simulink model "CF016A_GmVehSpdArbn"  (R2013b)
settings: Solver=FixedStepDiscrete  SolverMode=SingleTasking  StartTime=0.0  StopTime=1  FixedStep=0.002  RelTol=1e-3
undefined symbols (not defined in the file): DIAGCSTRTUPDLY_CNT_U32, NODEBSTEP_CNT_U16, NtcNr1, NtcSts1, VEHSPDMAX_KPH_F32
libraries: simulink x8, NxtrMax x7, NxtrMin x3, NxtrLim x3
(part 3 of 5)

== system CF016A_GmVehSpdArbn/GmVehSpdArbn/GmVehSpdArbnPer1/Calc_NTCIdleTi ==
  Constant1 : Constant  Value=DIAGCSTRTUPDLY_CNT_U32  OutDataTypeStr=uint32
  CopyRight2 : Subsystem  Description=|  mask(Copyright Information){none=on}
      | Copyright info block.                                               
      |                                                                     
      | Place copyright information at the top of every subsystem in design.
      mask prompts: none "No parameters"
      mask help: Place copyright information at the top of every subsystem in design.
      mask Display:
      | NxtrConf = 'Nexteer Confidential';
      | 
      | sys = bdroot; %handle for the current model ("system")
      | first = get_param(sys,'Created');
      | if(isempty(first))
      |     first = datestr(now,'yyyy');
      | else
      |     first = first(end-3:end);  %year is last four digits
      | end
      | 
      | last = get_param(sys,'LastModifiedDate');
      | if isempty(last)
      |     last = datestr(now,'yyyy');
      | else
      |     last = last(end-3:end);
      | end
      | 
      | if strcmp(first,last)
      |     fprintf('%s -- Copyright %s Nexteer',NxtrConf,first)
      | else
      |     fprintf('%s -- %s%s- %s Nexteer',NxtrConf,char(169),first,last)
      | end
  Data Store Read2 : DataStoreRead  DataStoreName=DiagcRefTi
  GetTiSpan100MicroSec32bit : Subsystem
  Relational Operator2 : RelationalOperator  Operator=>  OutDataTypeStr=boolean
  NTCIdleTiPassd : Outport
  wires:
  Constant1/1 -> Relational Operator2/2
  Relational Operator2/1 -> NTCIdleTiPassd/1  "NTCIdleTiPassd_Cnt_T_logl"
  Data Store Read2/1 -> GetTiSpan100MicroSec32bit/1(RefTmr)
  GetTiSpan100MicroSec32bit/1(TiSpan) -> Relational Operator2/1

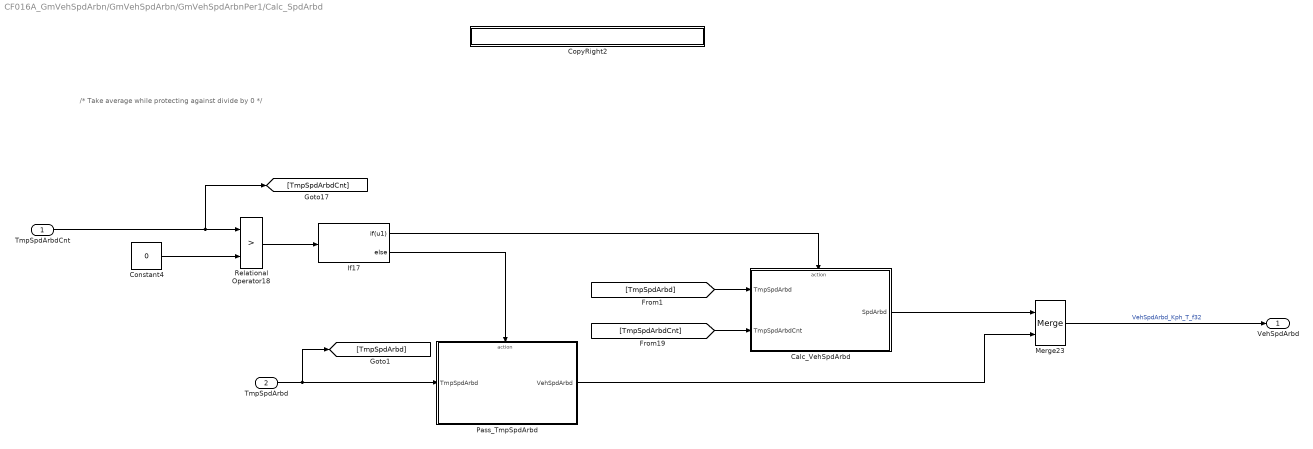
== system CF016A_GmVehSpdArbn/GmVehSpdArbn/GmVehSpdArbnPer1/Calc_SpdArbd ==
  note: /* Take average while protecting against divide by 0 */
  TmpSpdArbdCnt : Inport
  TmpSpdArbd : Inport  Port=2
  Calc_VehSpdArbd : Subsystem  TreatAsAtomicUnit=on
  Constant4 : Constant  Value=0  OutDataTypeStr=single
      settings: AttributesFormatString=%<OutDataTypeStr>
  CopyRight2 : Subsystem  Description=|  mask(Copyright Information){none=on}
      | Copyright info block.                                               
      |                                                                     
      | Place copyright information at the top of every subsystem in design.
      mask prompts: none "No parameters"
      mask help: Place copyright information at the top of every subsystem in design.
      mask Display:
      | NxtrConf = 'Nexteer Confidential';
      | 
      | sys = bdroot; %handle for the current model ("system")
      | first = get_param(sys,'Created');
      | if(isempty(first))
      |     first = datestr(now,'yyyy');
      | else
      |     first = first(end-3:end);  %year is last four digits
      | end
      | 
      | last = get_param(sys,'LastModifiedDate');
      | if isempty(last)
      |     last = datestr(now,'yyyy');
      | else
      |     last = last(end-3:end);
      | end
      | 
      | if strcmp(first,last)
      |     fprintf('%s -- Copyright %s Nexteer',NxtrConf,first)
      | else
      |     fprintf('%s -- %s%s- %s Nexteer',NxtrConf,char(169),first,last)
      | end
  If17 : If  IfExpression=u1
      settings: AttributesFormatString=%<Priority>
  Merge23 : Merge
  Pass_TmpSpdArbd : Subsystem  TreatAsAtomicUnit=on
  Relational Operator18 : RelationalOperator  Operator=>  OutDataTypeStr=boolean
  VehSpdArbd : Outport
  wires:
  Constant4/1 -> Relational Operator18/2
  Relational Operator18/1 -> If17/1
  If17/1 -> Calc_VehSpdArbd/Action
  If17/2 -> Pass_TmpSpdArbd/Action
  Pass_TmpSpdArbd/1(VehSpdArbd) -> Merge23/2
  Calc_VehSpdArbd/1(SpdArbd) -> Merge23/1
  Merge23/1 -> VehSpdArbd/1  "VehSpdArbd_Kph_T_f32"
  TmpSpdArbdCnt/1 -> [TmpSpdArbdCnt], Relational Operator18/1
  [TmpSpdArbdCnt] -> Calc_VehSpdArbd/2(TmpSpdArbdCnt)
  TmpSpdArbd/1 -> Pass_TmpSpdArbd/1(TmpSpdArbd), [TmpSpdArbd]
  [TmpSpdArbd] -> Calc_VehSpdArbd/1(TmpSpdArbd)

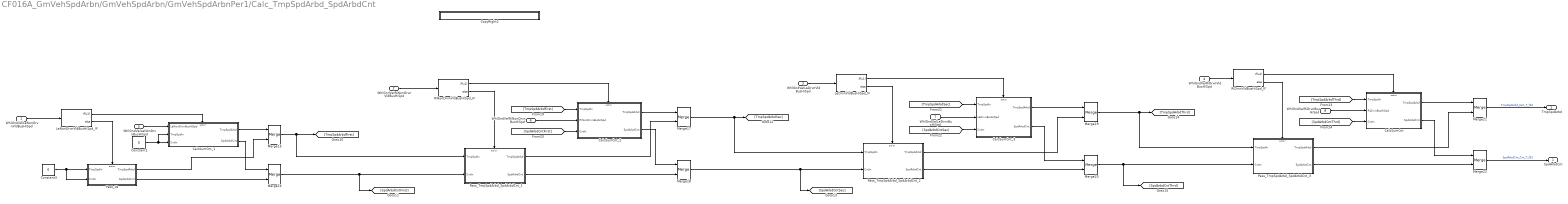
== system CF016A_GmVehSpdArbn/GmVehSpdArbn/GmVehSpdArbnPer1/Calc_TmpSpdArbd_SpdArbdCnt ==
  WhlGndVelLeNonDrvnVldBusHiSpd : Inport
  WhlGndVelRiNonDrvnVldBusHiSpd : Inport  RequirementInfo="{'linktype_rmi_doors' '0000c6e6 (/GM T1XX/SubSystem Specifications/Customer Functions/CF016A GM Vehicle Speed Arbitration)' '#197' 'true' 'REQ:  197' '' } %GIDa_75a6d6cd_4173_4b94_b70a_dd22fcf6fc32"  Port=2
  WhlGndVelLeDrvnVldBusHiSpd : Inport  RequirementInfo="{'linktype_rmi_doors' '0000c6e6 (/GM T1XX/SubSystem Specifications/Customer Functions/CF016A GM Vehicle Speed Arbitration)' '#197' 'true' 'REQ:  197' '' } %GIDa_bba5e7ef_449f_44f6_98d0_1ccf08468637"  Port=3
  WhlGndVelRiDrvnVldBusHiSpd : Inport  RequirementInfo="{'linktype_rmi_doors' '0000c6e6 (/GM T1XX/SubSystem Specifications/Customer Functions/CF016A GM Vehicle Speed Arbitration)' '#197' 'true' 'REQ:  197' '' } %GIDa_b5b50655_d2e5_4a4e_9d9c_e6104a63ae0b"  Port=4
  WhlGndVelLeNonDrvnBusHiSpd : Inport  RequirementInfo="{'linktype_rmi_doors' '0000c6e6 (/GM T1XX/SubSystem Specifications/Customer Functions/CF016A GM Vehicle Speed Arbitration)' '#197' 'true' 'REQ:  197' '' } %GIDa_3165a49e_7db2_44a5_86aa_6dde81cf1a65"  Port=5
  WhlGndVelRiNonDrvnBusHiSpd : Inport  RequirementInfo="{'linktype_rmi_doors' '0000c6e6 (/GM T1XX/SubSystem Specifications/Customer Functions/CF016A GM Vehicle Speed Arbitration)' '#197' 'true' 'REQ:  197' '' } %GIDa_3798149f_5af7_41c0_afc1_7eafa55e1dcf"  Port=6
  WhlGndVelLeDrvnBusHiSpd : Inport  RequirementInfo="{'linktype_rmi_doors' '0000c6e6 (/GM T1XX/SubSystem Specifications/Customer Functions/CF016A GM Vehicle Speed Arbitration)' '#197' 'true' 'REQ:  197' '' } %GIDa_8f8a555f_8d7e_4f96_a446_1dcec9e14b78"  Port=7
  WhlGndVelRiDrvnBusHiSpd : Inport  RequirementInfo="{'linktype_rmi_doors' '0000c6e6 (/GM T1XX/SubSystem Specifications/Customer Functions/CF016A GM Vehicle Speed Arbitration)' '#197' 'true' 'REQ:  197' '' } %GIDa_00fa1cd6_a6a5_410d_9383_797401eb3683"  Port=8
  CalcSumCnt : Subsystem  RequirementInfo="{'linktype_rmi_doors' '0000c6e6 (/GM T1XX/SubSystem Specifications/Customer Functions/CF016A GM Vehicle Speed Arbitration)' '#197' 'true' 'REQ:  197' '' } %GIDa_a224d60f_a880_4ee1_8319_45ce552737be"  TreatAsAtomicUnit=on
  CalcSumCnt_1 : Subsystem  RequirementInfo="{'linktype_rmi_doors' '0000c6e6 (/GM T1XX/SubSystem Specifications/Customer Functions/CF016A GM Vehicle Speed Arbitration)' '#197' 'true' 'REQ:  197' '' } %GIDa_a912f7bd_e18e_48b0_96ea_183fa55b44d1"  TreatAsAtomicUnit=on
  CalcSumCnt_2 : Subsystem  RequirementInfo="{'linktype_rmi_doors' '0000c6e6 (/GM T1XX/SubSystem Specifications/Customer Functions/CF016A GM Vehicle Speed Arbitration)' '#197' 'true' 'REQ:  197' '' } %GIDa_908d3886_164f_47bf_8eb5_d3c275cb63fb"  TreatAsAtomicUnit=on
  CalcSumCnt_3 : Subsystem  RequirementInfo="{'linktype_rmi_doors' '0000c6e6 (/GM T1XX/SubSystem Specifications/Customer Functions/CF016A GM Vehicle Speed Arbitration)' '#197' 'true' 'REQ:  197' '' } %GIDa_0cfda85e_115e_4a3a_86a7_df581f2b4836"  TreatAsAtomicUnit=on
  Constant1 : Constant  Value=0  OutDataTypeStr=single
      settings: AttributesFormatString=%<OutDataTypeStr>
  Constant3 : Constant  Value=0  OutDataTypeStr=single
      settings: AttributesFormatString=%<OutDataTypeStr>
  CopyRight2 : Subsystem  Description=|  mask(Copyright Information){none=on}
      | Copyright info block.                                               
      |                                                                     
      | Place copyright information at the top of every subsystem in design.
      mask prompts: none "No parameters"
      mask help: Place copyright information at the top of every subsystem in design.
      mask Display:
      | NxtrConf = 'Nexteer Confidential';
      | 
      | sys = bdroot; %handle for the current model ("system")
      | first = get_param(sys,'Created');
      | if(isempty(first))
      |     first = datestr(now,'yyyy');
      | else
      |     first = first(end-3:end);  %year is last four digits
      | end
      | 
      | last = get_param(sys,'LastModifiedDate');
      | if isempty(last)
      |     last = datestr(now,'yyyy');
      | else
      |     last = last(end-3:end);
      | end
      | 
      | if strcmp(first,last)
      |     fprintf('%s -- Copyright %s Nexteer',NxtrConf,first)
      | else
      |     fprintf('%s -- %s%s- %s Nexteer',NxtrConf,char(169),first,last)
      | end
  LeDrvnVldBusHiSpd_IF : If  RequirementInfo="{'linktype_rmi_doors' '0000c6e6 (/GM T1XX/SubSystem Specifications/Customer Functions/CF016A GM Vehicle Speed Arbitration)' '#197' 'true' 'REQ:  197' '' } %GIDa_e5398537_68ff_4ca3_873a_5860dedb4f38"  IfExpression=u1
      settings: AttributesFormatString=%<Priority>
  LeNonDrvnVldBusHiSpd_IF : If  RequirementInfo="{'linktype_rmi_doors' '0000c6e6 (/GM T1XX/SubSystem Specifications/Customer Functions/CF016A GM Vehicle Speed Arbitration)' '#197' 'true' 'REQ:  197' '' } %GIDa_0a5ef933_02c3_4017_8cbc_cbbf00c96bdb"  IfExpression=u1
      settings: AttributesFormatString=%<Priority>
  Merge15 : Merge  RequirementInfo="{'linktype_rmi_doors' '0000c6e6 (/GM T1XX/SubSystem Specifications/Customer Functions/CF016A GM Vehicle Speed Arbitration)' '#197' 'true' 'REQ:  197' '' } %GIDa_b01b27b6_2653_40db_b669_b9a443f48c3f"
  Merge16 : Merge  RequirementInfo="{'linktype_rmi_doors' '0000c6e6 (/GM T1XX/SubSystem Specifications/Customer Functions/CF016A GM Vehicle Speed Arbitration)' '#197' 'true' 'REQ:  197' '' } %GIDa_8a935c09_276b_472e_be93_82eb8a41092d"
  Merge17 : Merge  RequirementInfo="{'linktype_rmi_doors' '0000c6e6 (/GM T1XX/SubSystem Specifications/Customer Functions/CF016A GM Vehicle Speed Arbitration)' '#197' 'true' 'REQ:  197' '' } %GIDa_1a065b5b_19d5_4f28_8260_459213537fb4"
  Merge18 : Merge  RequirementInfo="{'linktype_rmi_doors' '0000c6e6 (/GM T1XX/SubSystem Specifications/Customer Functions/CF016A GM Vehicle Speed Arbitration)' '#197' 'true' 'REQ:  197' '' } %GIDa_74f763ca_8a5c_4a42_8005_2c77b166578e"
  Merge19 : Merge  RequirementInfo="{'linktype_rmi_doors' '0000c6e6 (/GM T1XX/SubSystem Specifications/Customer Functions/CF016A GM Vehicle Speed Arbitration)' '#197' 'true' 'REQ:  197' '' } %GIDa_3ff2a4ad_b1a8_4288_966c_4fbb914ab0f1"
  Merge20 : Merge  RequirementInfo="{'linktype_rmi_doors' '0000c6e6 (/GM T1XX/SubSystem Specifications/Customer Functions/CF016A GM Vehicle Speed Arbitration)' '#197' 'true' 'REQ:  197' '' } %GIDa_5cafa504_1ff8_4f3c_b0c4_59e13f736e29"
  Merge21 : Merge  RequirementInfo="{'linktype_rmi_doors' '0000c6e6 (/GM T1XX/SubSystem Specifications/Customer Functions/CF016A GM Vehicle Speed Arbitration)' '#197' 'true' 'REQ:  197' '' } %GIDa_e6f4a7a3_924e_49ec_a51b_ec7f1402c916"
  Merge22 : Merge  RequirementInfo="{'linktype_rmi_doors' '0000c6e6 (/GM T1XX/SubSystem Specifications/Customer Functions/CF016A GM Vehicle Speed Arbitration)' '#197' 'true' 'REQ:  197' '' } %GIDa_5f365e82_5eef_48d0_8df9_073c5a4821ae"
  Pass_0s : Subsystem  RequirementInfo="{'linktype_rmi_doors' '0000c6e6 (/GM T1XX/SubSystem Specifications/Customer Functions/CF016A GM Vehicle Speed Arbitration)' '#197' 'true' 'REQ:  197' '' } %GIDa_d72c6e09_db59_44fd_869f_4f3454a9c428"  TreatAsAtomicUnit=on
  Pass_TmpSpdArbd_SpdArbdCnt_1 : Subsystem  RequirementInfo="{'linktype_rmi_doors' '0000c6e6 (/GM T1XX/SubSystem Specifications/Customer Functions/CF016A GM Vehicle Speed Arbitration)' '#197' 'true' 'REQ:  197' '' } %GIDa_b9dcaff2_4061_4b5b_a6b9_7f9acd096b10"  TreatAsAtomicUnit=on
  Pass_TmpSpdArbd_SpdArbdCnt_2 : Subsystem  RequirementInfo="{'linktype_rmi_doors' '0000c6e6 (/GM T1XX/SubSystem Specifications/Customer Functions/CF016A GM Vehicle Speed Arbitration)' '#197' 'true' 'REQ:  197' '' } %GIDa_23d3c945_9e72_4aec_902a_23e89c0b8921"  TreatAsAtomicUnit=on
  Pass_TmpSpdArbd_SpdArbdCnt_3 : Subsystem  RequirementInfo="{'linktype_rmi_doors' '0000c6e6 (/GM T1XX/SubSystem Specifications/Customer Functions/CF016A GM Vehicle Speed Arbitration)' '#197' 'true' 'REQ:  197' '' } %GIDa_e40d34b4_e19b_484e_8b3e_f03258be8dd4"  TreatAsAtomicUnit=on
  RiDrvnVldBusHiSpd_IF : If  RequirementInfo="{'linktype_rmi_doors' '0000c6e6 (/GM T1XX/SubSystem Specifications/Customer Functions/CF016A GM Vehicle Speed Arbitration)' '#197' 'true' 'REQ:  197' '' } %GIDa_4ee12af2_8377_4892_bcba_172ca4ea6a57"  IfExpression=u1
      settings: AttributesFormatString=%<Priority>
  RiNonDrvnVldBusHiSpd_IF : If  RequirementInfo="{'linktype_rmi_doors' '0000c6e6 (/GM T1XX/SubSystem Specifications/Customer Functions/CF016A GM Vehicle Speed Arbitration)' '#197' 'true' 'REQ:  197' '' } %GIDa_85933de9_8d8e_4fbe_a57f_f54c76ec7632"  IfExpression=u1
      settings: AttributesFormatString=%<Priority>
  SpdArbdCnt : Outport  RequirementInfo="{'linktype_rmi_doors' '0000c6e6 (/GM T1XX/SubSystem Specifications/Customer Functions/CF016A GM Vehicle Speed Arbitration)' '#197' 'true' 'REQ:  197' '' } %GIDa_e429be63_e02c_47c7_b0ac_69f68d853113"
  TmpSpdArbd : Outport  RequirementInfo="{'linktype_rmi_doors' '0000c6e6 (/GM T1XX/SubSystem Specifications/Customer Functions/CF016A GM Vehicle Speed Arbitration)' '#197' 'true' 'REQ:  197' '' } %GIDa_84bb4a95_512d_415c_8720_8fa48f017119"  Port=2
  wires:
  LeNonDrvnVldBusHiSpd_IF/1 -> CalcSumCnt_1/Action
  LeNonDrvnVldBusHiSpd_IF/2 -> Pass_0s/Action
  CalcSumCnt_1/1(TmpSpdArbd) -> Merge15/1
  Pass_0s/1(TmpSpdArbd) -> Merge15/2
  Merge15/1 -> [TmpSpdArbdFirst], Pass_TmpSpdArbd_SpdArbdCnt_1/1(TmpSpdIn)
  Pass_0s/2(SpdArbdCnt) -> Merge16/2
  CalcSumCnt_1/2(SpdArbdCnt) -> Merge16/1
  Merge16/1 -> [SpdArbdCntFirst], Pass_TmpSpdArbd_SpdArbdCnt_1/2(CntIn)
  RiNonDrvnVldBusHiSpd_IF/1 -> CalcSumCnt_2/Action
  RiNonDrvnVldBusHiSpd_IF/2 -> Pass_TmpSpdArbd_SpdArbdCnt_1/Action
  CalcSumCnt_2/1(TmpSpdArbd) -> Merge17/1
  Pass_TmpSpdArbd_SpdArbdCnt_1/1(TmpSpdArbd) -> Merge17/2
  Pass_TmpSpdArbd_SpdArbdCnt_1/2(SpdArbdCnt) -> Merge18/2
  CalcSumCnt_2/2(SpdArbdCnt) -> Merge18/1
  WhlGndVelRiNonDrvnBusHiSpd/1 -> CalcSumCnt_2/2(RiNonDrvnBusHiSpd)
  [TmpSpdArbdFirst] -> CalcSumCnt_2/1(TmpSpdIn)
  [SpdArbdCntFirst] -> CalcSumCnt_2/3(CntIn)
  Merge17/1 -> [TmpSpdArbdSec], Pass_TmpSpdArbd_SpdArbdCnt_2/1(TmpSpdIn)
  LeDrvnVldBusHiSpd_IF/1 -> CalcSumCnt_3/Action
  LeDrvnVldBusHiSpd_IF/2 -> Pass_TmpSpdArbd_SpdArbdCnt_2/Action
  Pass_TmpSpdArbd_SpdArbdCnt_2/1(TmpSpdArbd) -> Merge19/2
  Pass_TmpSpdArbd_SpdArbdCnt_2/2(SpdArbdCnt) -> Merge20/2
  WhlGndVelLeDrvnBusHiSpd/1 -> CalcSumCnt_3/2(LeDrvnBusHiSpd)
  [TmpSpdArbdSec] -> CalcSumCnt_3/1(TmpSpdIn)
  [SpdArbdCntSec] -> CalcSumCnt_3/3(CntIn)
  CalcSumCnt_3/1(TmpSpdArbd) -> Merge19/1
  CalcSumCnt_3/2(SpdArbdCnt) -> Merge20/1
  Merge19/1 -> Pass_TmpSpdArbd_SpdArbdCnt_3/1(TmpSpdIn), [TmpSpdArbdThrd]
  RiDrvnVldBusHiSpd_IF/1 -> CalcSumCnt/Action
  RiDrvnVldBusHiSpd_IF/2 -> Pass_TmpSpdArbd_SpdArbdCnt_3/Action
  Pass_TmpSpdArbd_SpdArbdCnt_3/1(TmpSpdArbd) -> Merge21/2
  Pass_TmpSpdArbd_SpdArbdCnt_3/2(SpdArbdCnt) -> Merge22/2
  WhlGndVelRiDrvnBusHiSpd/1 -> CalcSumCnt/2(RiDrvnBusHiSpd)
  [TmpSpdArbdThrd] -> CalcSumCnt/1(TmpSpdIn)
  [SpdArbdCntThrd] -> CalcSumCnt/3(CntIn)
  CalcSumCnt/1(TmpSpdArbd) -> Merge21/1
  CalcSumCnt/2(SpdArbdCnt) -> Merge22/1
  Merge18/1 -> [SpdArbdCntSec], Pass_TmpSpdArbd_SpdArbdCnt_2/2(CntIn)
  Merge20/1 -> [SpdArbdCntThrd], Pass_TmpSpdArbd_SpdArbdCnt_3/2(CntIn)
  Merge21/1 -> TmpSpdArbd/1  "TmpSpdArbd_Kph_T_f32"
  Merge22/1 -> SpdArbdCnt/1  "SpdArbdCnt_Cnt_T_f32"
  WhlGndVelRiNonDrvnVldBusHiSpd/1 -> RiNonDrvnVldBusHiSpd_IF/1
  WhlGndVelLeDrvnVldBusHiSpd/1 -> LeDrvnVldBusHiSpd_IF/1
  WhlGndVelLeNonDrvnBusHiSpd/1 -> CalcSumCnt_1/1(LeNonDrvnBusHiSpd)
  WhlGndVelRiDrvnVldBusHiSpd/1 -> RiDrvnVldBusHiSpd_IF/1
  WhlGndVelLeNonDrvnVldBusHiSpd/1 -> LeNonDrvnVldBusHiSpd_IF/1
  Constant3/1 -> Pass_0s/2(CntIn), Pass_0s/1(TmpSpdIn)
  Constant1/1 -> CalcSumCnt_1/3(CntIn), CalcSumCnt_1/2(TmpSpdIn)

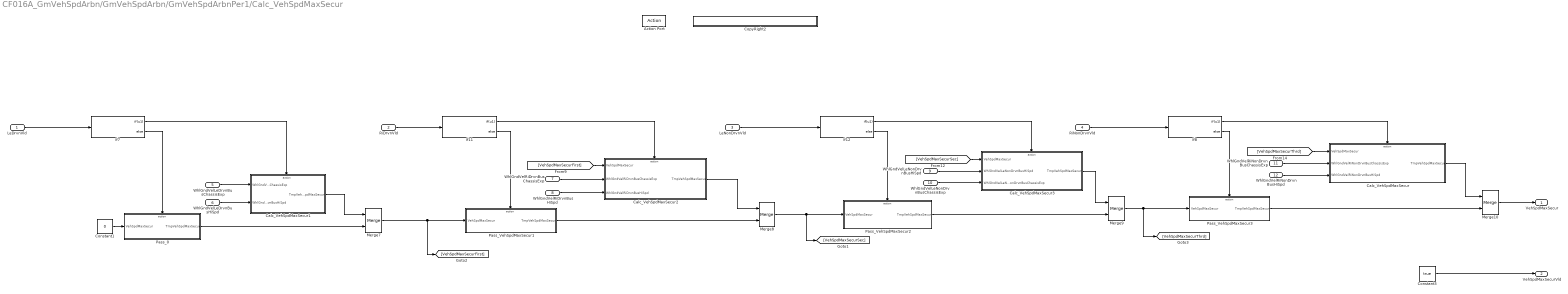
== system CF016A_GmVehSpdArbn/GmVehSpdArbn/GmVehSpdArbnPer1/Calc_VehSpdMaxSecur ==
  LeDrvnVld : Inport  RequirementInfo="{'linktype_rmi_doors' '0000c6e6 (/GM T1XX/SubSystem Specifications/Customer Functions/CF016A GM Vehicle Speed Arbitration)' '#191' 'true' 'REQ:  191' '' } %GIDa_016e9a8c_0dee_441f_b371_be7f32efee97"
  RiDrvnVld : Inport  RequirementInfo="{'linktype_rmi_doors' '0000c6e6 (/GM T1XX/SubSystem Specifications/Customer Functions/CF016A GM Vehicle Speed Arbitration)' '#191' 'true' 'REQ:  191' '' } %GIDa_128bb698_b54e_4ac3_804e_c7544f2786d8"  Port=2  OutDataTypeStr=boolean
  LeNonDrvnVld : Inport  RequirementInfo="{'linktype_rmi_doors' '0000c6e6 (/GM T1XX/SubSystem Specifications/Customer Functions/CF016A GM Vehicle Speed Arbitration)' '#191' 'true' 'REQ:  191' '' } %GIDa_acbf9984_1b4c_419e_9dcc_bea34cf10fd2"  Port=3  OutDataTypeStr=boolean
  RiNonDrvnVld : Inport  RequirementInfo="{'linktype_rmi_doors' '0000c6e6 (/GM T1XX/SubSystem Specifications/Customer Functions/CF016A GM Vehicle Speed Arbitration)' '#191' 'true' 'REQ:  191' '' } %GIDa_25ad80e8_ae7b_4422_af9f_de8db34a4b72"  Port=4  OutDataTypeStr=boolean
  WhlGndVelLeDrvnBusChassisExp : Inport  RequirementInfo="{'linktype_rmi_doors' '0000c6e6 (/GM T1XX/SubSystem Specifications/Customer Functions/CF016A GM Vehicle Speed Arbitration)' '#191' 'true' 'REQ:  191' '' } %GIDa_6478f328_db51_4002_ad33_9728e1be5be7"  Port=5
  WhlGndVelLeDrvnBusHiSpd : Inport  RequirementInfo="{'linktype_rmi_doors' '0000c6e6 (/GM T1XX/SubSystem Specifications/Customer Functions/CF016A GM Vehicle Speed Arbitration)' '#191' 'true' 'REQ:  191' '' } %GIDa_9d10f7bb_bd83_4311_b6a9_b26e37384eaf"  Port=6
  WhlGndVelRiDrvnBusChassisExp : Inport  RequirementInfo="{'linktype_rmi_doors' '0000c6e6 (/GM T1XX/SubSystem Specifications/Customer Functions/CF016A GM Vehicle Speed Arbitration)' '#191' 'true' 'REQ:  191' '' } %GIDa_2cb3bc06_4ce5_4f44_8592_3e983cb75be4"  Port=7
  WhlGndVelRiDrvnBusHiSpd : Inport  RequirementInfo="{'linktype_rmi_doors' '0000c6e6 (/GM T1XX/SubSystem Specifications/Customer Functions/CF016A GM Vehicle Speed Arbitration)' '#191' 'true' 'REQ:  191' '' } %GIDa_3229f93c_7f8a_49f2_a195_27dc770874c0"  Port=8
  WhlGndVelLeNonDrvnBusHiSpd : Inport  RequirementInfo="{'linktype_rmi_doors' '0000c6e6 (/GM T1XX/SubSystem Specifications/Customer Functions/CF016A GM Vehicle Speed Arbitration)' '#191' 'true' 'REQ:  191' '' } %GIDa_3da011a6_c346_4167_8828_605637927bbd"  Port=9
  WhlGndVelLeNonDrvnBusChassisExp : Inport  RequirementInfo="{'linktype_rmi_doors' '0000c6e6 (/GM T1XX/SubSystem Specifications/Customer Functions/CF016A GM Vehicle Speed Arbitration)' '#191' 'true' 'REQ:  191' '' } %GIDa_9b07bb93_0a24_48a3_9ef8_ce51cbd8d5c9"  Port=10
  WhlGndVelRiNonDrvnBusChassisExp : Inport  RequirementInfo="{'linktype_rmi_doors' '0000c6e6 (/GM T1XX/SubSystem Specifications/Customer Functions/CF016A GM Vehicle Speed Arbitration)' '#191' 'true' 'REQ:  191' '' } %GIDa_3388bfa8_e61d_4eed_84f0_18253f8ee8d4"  Port=11
  WhlGndVelRiNonDrvnBusHiSpd : Inport  RequirementInfo="{'linktype_rmi_doors' '0000c6e6 (/GM T1XX/SubSystem Specifications/Customer Functions/CF016A GM Vehicle Speed Arbitration)' '#191' 'true' 'REQ:  191' '' } %GIDa_3473fc1e_ce6d_4e03_beb3_66a3ec9a4f7d"  Port=12
  Action Port : ActionPort  ActionType=else
  Calc_VehSpdMaxSecur : Subsystem  RequirementInfo="{'linktype_rmi_doors' '0000c6e6 (/GM T1XX/SubSystem Specifications/Customer Functions/CF016A GM Vehicle Speed Arbitration)' '#191' 'true' 'REQ:  191' '' } %GIDa_aa0d8ce0_0107_46c0_b257_d6af669a8052"  TreatAsAtomicUnit=on
  Calc_VehSpdMaxSecur1 : Subsystem  RequirementInfo="{'linktype_rmi_doors' '0000c6e6 (/GM T1XX/SubSystem Specifications/Customer Functions/CF016A GM Vehicle Speed Arbitration)' '#191' 'true' 'REQ:  191' '' } %GIDa_613ec262_9660_483f_a2f3_f3d5c6300cd4"  TreatAsAtomicUnit=on
  Calc_VehSpdMaxSecur2 : Subsystem  RequirementInfo="{'linktype_rmi_doors' '0000c6e6 (/GM T1XX/SubSystem Specifications/Customer Functions/CF016A GM Vehicle Speed Arbitration)' '#191' 'true' 'REQ:  191' '' } %GIDa_0c7a7f52_37f4_4b29_bcff_3befa50c22fb"  TreatAsAtomicUnit=on
  Calc_VehSpdMaxSecur3 : Subsystem  RequirementInfo="{'linktype_rmi_doors' '0000c6e6 (/GM T1XX/SubSystem Specifications/Customer Functions/CF016A GM Vehicle Speed Arbitration)' '#191' 'true' 'REQ:  191' '' } %GIDa_c073966b_de96_409c_93ca_f5f33421aedd"  TreatAsAtomicUnit=on
  Constant1 : Constant  Value=0  OutDataTypeStr=single
      settings: AttributesFormatString=%<OutDataTypeStr>
  Constant3 : Constant  RequirementInfo="{'linktype_rmi_doors' '0000c6e6 (/GM T1XX/SubSystem Specifications/Customer Functions/CF016A GM Vehicle Speed Arbitration)' '#151' 'true' 'REQ:  151' '' } %GIDa_7e2fc1cc_2834_44bc_ad76_c37ac143b7f7"  Value=true  OutDataTypeStr=boolean
      settings: AttributesFormatString=%<OutDataTypeStr>
  CopyRight2 : Subsystem  Description=|  mask(Copyright Information){none=on}
      | Copyright info block.                                               
      |                                                                     
      | Place copyright information at the top of every subsystem in design.
      mask prompts: none "No parameters"
      mask help: Place copyright information at the top of every subsystem in design.
      mask Display:
      | NxtrConf = 'Nexteer Confidential';
      | 
      | sys = bdroot; %handle for the current model ("system")
      | first = get_param(sys,'Created');
      | if(isempty(first))
      |     first = datestr(now,'yyyy');
      | else
      |     first = first(end-3:end);  %year is last four digits
      | end
      | 
      | last = get_param(sys,'LastModifiedDate');
      | if isempty(last)
      |     last = datestr(now,'yyyy');
      | else
      |     last = last(end-3:end);
      | end
      | 
      | if strcmp(first,last)
      |     fprintf('%s -- Copyright %s Nexteer',NxtrConf,first)
      | else
      |     fprintf('%s -- %s%s- %s Nexteer',NxtrConf,char(169),first,last)
      | end
  If11 : If  RequirementInfo="{'linktype_rmi_doors' '0000c6e6 (/GM T1XX/SubSystem Specifications/Customer Functions/CF016A GM Vehicle Speed Arbitration)' '#191' 'true' 'REQ:  191' '' } %GIDa_3b960e7e_430b_4cee_846e_0c086220ad1d"  IfExpression=u1
      settings: AttributesFormatString=%<Priority>
  If12 : If  RequirementInfo="{'linktype_rmi_doors' '0000c6e6 (/GM T1XX/SubSystem Specifications/Customer Functions/CF016A GM Vehicle Speed Arbitration)' '#191' 'true' 'REQ:  191' '' } %GIDa_b4134c6a_61c4_4593_881c_74b2ea1a1309"  IfExpression=u1
      settings: AttributesFormatString=%<Priority>
  If7 : If  RequirementInfo="{'linktype_rmi_doors' '0000c6e6 (/GM T1XX/SubSystem Specifications/Customer Functions/CF016A GM Vehicle Speed Arbitration)' '#191' 'true' 'REQ:  191' '' } %GIDa_0c2f14b7_51fd_4b78_9785_f168a14d3cb2"  IfExpression=u1
      settings: AttributesFormatString=%<Priority>
  If8 : If  RequirementInfo="{'linktype_rmi_doors' '0000c6e6 (/GM T1XX/SubSystem Specifications/Customer Functions/CF016A GM Vehicle Speed Arbitration)' '#191' 'true' 'REQ:  191' '' } %GIDa_aea6c2b9_e571_43da_b054_95cf4e8d3382"  IfExpression=u1
      settings: AttributesFormatString=%<Priority>
  Merge10 : Merge  RequirementInfo="{'linktype_rmi_doors' '0000c6e6 (/GM T1XX/SubSystem Specifications/Customer Functions/CF016A GM Vehicle Speed Arbitration)' '#191' 'true' 'REQ:  191' '' } %GIDa_f63e1bcc_f9f1_4715_bb8c_bbaac44b742d"
  Merge7 : Merge  RequirementInfo="{'linktype_rmi_doors' '0000c6e6 (/GM T1XX/SubSystem Specifications/Customer Functions/CF016A GM Vehicle Speed Arbitration)' '#191' 'true' 'REQ:  191' '' } %GIDa_630989c1_0d1e_45b2_bb4d_1ad3f01457a0"
  Merge8 : Merge  RequirementInfo="{'linktype_rmi_doors' '0000c6e6 (/GM T1XX/SubSystem Specifications/Customer Functions/CF016A GM Vehicle Speed Arbitration)' '#191' 'true' 'REQ:  191' '' } %GIDa_69cca6fe_27ca_4fae_938b_6763fc777559"
  Merge9 : Merge  RequirementInfo="{'linktype_rmi_doors' '0000c6e6 (/GM T1XX/SubSystem Specifications/Customer Functions/CF016A GM Vehicle Speed Arbitration)' '#191' 'true' 'REQ:  191' '' } %GIDa_0a4d8527_d260_4c92_a8b8_61d26a3d98ce"
  Pass_0 : Subsystem  RequirementInfo="{'linktype_rmi_doors' '0000c6e6 (/GM T1XX/SubSystem Specifications/Customer Functions/CF016A GM Vehicle Speed Arbitration)' '#191' 'true' 'REQ:  191' '' } %GIDa_7deb987c_9544_4301_887a_e76b868b178a"  TreatAsAtomicUnit=on
  Pass_VehSpdMaxSecur1 : Subsystem  RequirementInfo="{'linktype_rmi_doors' '0000c6e6 (/GM T1XX/SubSystem Specifications/Customer Functions/CF016A GM Vehicle Speed Arbitration)' '#191' 'true' 'REQ:  191' '' } %GIDa_3f50bb7e_6f5f_433d_8a83_e591adaa77fe"  TreatAsAtomicUnit=on
  Pass_VehSpdMaxSecur2 : Subsystem  RequirementInfo="{'linktype_rmi_doors' '0000c6e6 (/GM T1XX/SubSystem Specifications/Customer Functions/CF016A GM Vehicle Speed Arbitration)' '#191' 'true' 'REQ:  191' '' } %GIDa_cc96ff68_da04_4f59_97f2_b30b80e13b50"  TreatAsAtomicUnit=on
  Pass_VehSpdMaxSecur3 : Subsystem  RequirementInfo="{'linktype_rmi_doors' '0000c6e6 (/GM T1XX/SubSystem Specifications/Customer Functions/CF016A GM Vehicle Speed Arbitration)' '#191' 'true' 'REQ:  191' '' } %GIDa_47dc531f_3549_46a1_ae9e_9f054f6e0236"  TreatAsAtomicUnit=on
  VehSpdMaxSecur : Outport  RequirementInfo="{'linktype_rmi_doors' '0000c6e6 (/GM T1XX/SubSystem Specifications/Customer Functions/CF016A GM Vehicle Speed Arbitration)' '#191' 'true' 'REQ:  191' '' } %GIDa_8971140d_7547_4d4d_b1e0_7bbf12f78ab4"
  VehSpdMaxSecurVld : Outport  RequirementInfo="{'linktype_rmi_doors' '0000c6e6 (/GM T1XX/SubSystem Specifications/Customer Functions/CF016A GM Vehicle Speed Arbitration)' '#151' 'true' 'REQ:  151' '' } %GIDa_e9b0385c_7d8a_4a1f_b12a_6635902ecd92"  Port=2
  wires:
  Constant3/1 -> VehSpdMaxSecurVld/1
  If7/1 -> Calc_VehSpdMaxSecur1/Action
  Calc_VehSpdMaxSecur1/1(TmpVehSpdMaxSecur) -> Merge7/1
  If7/2 -> Pass_0/Action
  Pass_0/1(TmpVehSpdMaxSecur) -> Merge7/2
  If11/1 -> Calc_VehSpdMaxSecur2/Action
  If11/2 -> Pass_VehSpdMaxSecur1/Action
  Pass_VehSpdMaxSecur1/1(TmpVehSpdMaxSecur) -> Merge8/2
  Calc_VehSpdMaxSecur2/1(TmpVehSpdMaxSecur) -> Merge8/1
  [VehSpdMaxSecurFirst] -> Calc_VehSpdMaxSecur2/1(VehSpdMaxSecur)
  If12/1 -> Calc_VehSpdMaxSecur3/Action
  If12/2 -> Pass_VehSpdMaxSecur2/Action
  Pass_VehSpdMaxSecur2/1(TmpVehSpdMaxSecur) -> Merge9/2
  Calc_VehSpdMaxSecur3/1(TmpVehSpdMaxSecur) -> Merge9/1
  [VehSpdMaxSecurSec] -> Calc_VehSpdMaxSecur3/1(VehSpdMaxSecur)
  If8/1 -> Calc_VehSpdMaxSecur/Action
  If8/2 -> Pass_VehSpdMaxSecur3/Action
  Pass_VehSpdMaxSecur3/1(TmpVehSpdMaxSecur) -> Merge10/2
  Calc_VehSpdMaxSecur/1(TmpVehSpdMaxSecur) -> Merge10/1
  [VehSpdMaxSecurThrd] -> Calc_VehSpdMaxSecur/1(VehSpdMaxSecur)
  Merge10/1 -> VehSpdMaxSecur/1
  WhlGndVelLeDrvnBusChassisExp/1 -> Calc_VehSpdMaxSecur1/1(WhlGndVelLeDrvnBusChassisExp)
  WhlGndVelLeDrvnBusHiSpd/1 -> Calc_VehSpdMaxSecur1/2(WhlGndVelLeDrvnBusHiSpd)
  WhlGndVelRiDrvnBusChassisExp/1 -> Calc_VehSpdMaxSecur2/2(WhlGndVelRiDrvnBusChassisExp)
  WhlGndVelRiDrvnBusHiSpd/1 -> Calc_VehSpdMaxSecur2/3(WhlGndVelRiDrvnBusHiSpd)
  WhlGndVelLeNonDrvnBusHiSpd/1 -> Calc_VehSpdMaxSecur3/2(WhlGndVelLeNonDrvnBusHiSpd)
  WhlGndVelLeNonDrvnBusChassisExp/1 -> Calc_VehSpdMaxSecur3/3(WhlGndVelLeNonDrvnBusChassisExp)
  WhlGndVelRiNonDrvnBusChassisExp/1 -> Calc_VehSpdMaxSecur/2(WhlGndVelRiNonDrvnBusChassisExp)
  WhlGndVelRiNonDrvnBusHiSpd/1 -> Calc_VehSpdMaxSecur/3(WhlGndVelRiNonDrvnBusHiSpd)
  Merge7/1 -> [VehSpdMaxSecurFirst], Pass_VehSpdMaxSecur1/1(VehSpdMaxSecur)
  Merge8/1 -> [VehSpdMaxSecurSec], Pass_VehSpdMaxSecur2/1(VehSpdMaxSecur)
  Merge9/1 -> [VehSpdMaxSecurThrd], Pass_VehSpdMaxSecur3/1(VehSpdMaxSecur)
  LeDrvnVld/1 -> If7/1
  RiNonDrvnVld/1 -> If8/1
  LeNonDrvnVld/1 -> If12/1
  RiDrvnVld/1 -> If11/1
  Constant1/1 -> Pass_0/1(VehSpdMaxSecur)

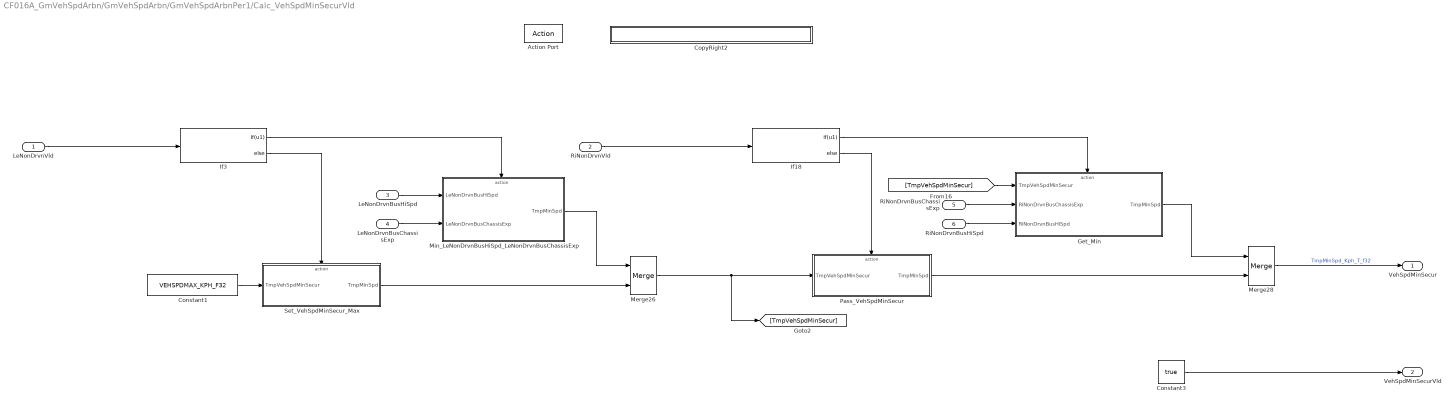
== system CF016A_GmVehSpdArbn/GmVehSpdArbn/GmVehSpdArbnPer1/Calc_VehSpdMinSecurVld ==
  LeNonDrvnVld : Inport  RequirementInfo="{'linktype_rmi_doors' '0000c6e6 (/GM T1XX/SubSystem Specifications/Customer Functions/CF016A GM Vehicle Speed Arbitration)' '#154' 'true' 'REQ:  154' '' } %GIDa_6d68e163_9d7b_4a2a_9a60_bdd96da40b8f"  OutDataTypeStr=boolean
  RiNonDrvnVld : Inport  RequirementInfo="{'linktype_rmi_doors' '0000c6e6 (/GM T1XX/SubSystem Specifications/Customer Functions/CF016A GM Vehicle Speed Arbitration)' '#154' 'true' 'REQ:  154' '' } %GIDa_fb21e64c_bd82_4709_a191_bd8baefcd19a"  Port=2  OutDataTypeStr=boolean
  LeNonDrvnBusHiSpd : Inport  RequirementInfo="{'linktype_rmi_doors' '0000c6e6 (/GM T1XX/SubSystem Specifications/Customer Functions/CF016A GM Vehicle Speed Arbitration)' '#154' 'true' 'REQ:  154' '' } %GIDa_a4cb8585_9b4a_430b_b664_a11d0feca6a8"  Port=3
  LeNonDrvnBusChassisExp : Inport  RequirementInfo="{'linktype_rmi_doors' '0000c6e6 (/GM T1XX/SubSystem Specifications/Customer Functions/CF016A GM Vehicle Speed Arbitration)' '#154' 'true' 'REQ:  154' '' } %GIDa_85fb64b9_775e_4475_8a0d_46047ecd73cf"  Port=4
  RiNonDrvnBusChassisExp : Inport  RequirementInfo="{'linktype_rmi_doors' '0000c6e6 (/GM T1XX/SubSystem Specifications/Customer Functions/CF016A GM Vehicle Speed Arbitration)' '#154' 'true' 'REQ:  154' '' } %GIDa_c2a4ed53_ebd4_4798_b198_c26d0f0fe646"  Port=5
  RiNonDrvnBusHiSpd : Inport  RequirementInfo="{'linktype_rmi_doors' '0000c6e6 (/GM T1XX/SubSystem Specifications/Customer Functions/CF016A GM Vehicle Speed Arbitration)' '#154' 'true' 'REQ:  154' '' } %GIDa_35ae5219_b5be_42e3_b723_156b85dd8673"  Port=6
  Action Port : ActionPort  ActionType=else
  Constant1 : Constant  Value=VEHSPDMAX_KPH_F32  OutDataTypeStr=single
      settings: AttributesFormatString=%<OutDataTypeStr>
  Constant3 : Constant  RequirementInfo="{'linktype_rmi_doors' '0000c6e6 (/GM T1XX/SubSystem Specifications/Customer Functions/CF016A GM Vehicle Speed Arbitration)' '#200' 'true' 'REQ:  200' '' } %GIDa_375dc1c7_f11c_4f5e_835d_549c189ff712"  Value=true  OutDataTypeStr=boolean
      settings: AttributesFormatString=%<OutDataTypeStr>
  CopyRight2 : Subsystem  Description=|  mask(Copyright Information){none=on}
      | Copyright info block.                                               
      |                                                                     
      | Place copyright information at the top of every subsystem in design.
      mask prompts: none "No parameters"
      mask help: Place copyright information at the top of every subsystem in design.
      mask Display:
      | NxtrConf = 'Nexteer Confidential';
      | 
      | sys = bdroot; %handle for the current model ("system")
      | first = get_param(sys,'Created');
      | if(isempty(first))
      |     first = datestr(now,'yyyy');
      | else
      |     first = first(end-3:end);  %year is last four digits
      | end
      | 
      | last = get_param(sys,'LastModifiedDate');
      | if isempty(last)
      |     last = datestr(now,'yyyy');
      | else
      |     last = last(end-3:end);
      | end
      | 
      | if strcmp(first,last)
      |     fprintf('%s -- Copyright %s Nexteer',NxtrConf,first)
      | else
      |     fprintf('%s -- %s%s- %s Nexteer',NxtrConf,char(169),first,last)
      | end
  Get_Min : Subsystem  RequirementInfo="{'linktype_rmi_doors' '0000c6e6 (/GM T1XX/SubSystem Specifications/Customer Functions/CF016A GM Vehicle Speed Arbitration)' '#154' 'true' 'REQ:  154' '' } %GIDa_d0b944f6_ff17_4739_ae27_f401cfc86d51"  TreatAsAtomicUnit=on
  If18 : If  RequirementInfo="{'linktype_rmi_doors' '0000c6e6 (/GM T1XX/SubSystem Specifications/Customer Functions/CF016A GM Vehicle Speed Arbitration)' '#154' 'true' 'REQ:  154' '' } %GIDa_5f607e3d_16f0_48ac_aa4b_3d0489ab76e6"  IfExpression=u1
      settings: AttributesFormatString=%<Priority>
  If3 : If  RequirementInfo="{'linktype_rmi_doors' '0000c6e6 (/GM T1XX/SubSystem Specifications/Customer Functions/CF016A GM Vehicle Speed Arbitration)' '#154' 'true' 'REQ:  154' '' } %GIDa_6366a054_c697_4421_90da_a84586a20777"  IfExpression=u1
      settings: AttributesFormatString=%<Priority>
  Merge26 : Merge  RequirementInfo="{'linktype_rmi_doors' '0000c6e6 (/GM T1XX/SubSystem Specifications/Customer Functions/CF016A GM Vehicle Speed Arbitration)' '#154' 'true' 'REQ:  154' '' } %GIDa_27859d07_7fd5_49b8_b06e_3d7852a073d0"
  Merge28 : Merge  RequirementInfo="{'linktype_rmi_doors' '0000c6e6 (/GM T1XX/SubSystem Specifications/Customer Functions/CF016A GM Vehicle Speed Arbitration)' '#154' 'true' 'REQ:  154' '' } %GIDa_fe027600_d924_4155_99c4_6c3a6becd523"
  Min_LeNonDrvnBusHiSpd_LeNonDrvnBusChassisExp : Subsystem  RequirementInfo="{'linktype_rmi_doors' '0000c6e6 (/GM T1XX/SubSystem Specifications/Customer Functions/CF016A GM Vehicle Speed Arbitration)' '#154' 'true' 'REQ:  154' '' } %GIDa_c99a0528_5b89_4885_a932_d7d2bb04fc4b"  TreatAsAtomicUnit=on
  Pass_VehSpdMinSecur : Subsystem  RequirementInfo="{'linktype_rmi_doors' '0000c6e6 (/GM T1XX/SubSystem Specifications/Customer Functions/CF016A GM Vehicle Speed Arbitration)' '#154' 'true' 'REQ:  154' '' } %GIDa_f01dd7ac_93c1_43fc_adb3_dea33215e594"  TreatAsAtomicUnit=on
  Set_VehSpdMinSecur_Max : Subsystem  RequirementInfo="{'linktype_rmi_doors' '0000c6e6 (/GM T1XX/SubSystem Specifications/Customer Functions/CF016A GM Vehicle Speed Arbitration)' '#154' 'true' 'REQ:  154' '' } %GIDa_20cb32d9_299e_45b6_8c43_31301e59aa06"  TreatAsAtomicUnit=on
  VehSpdMinSecur : Outport  RequirementInfo="{'linktype_rmi_doors' '0000c6e6 (/GM T1XX/SubSystem Specifications/Customer Functions/CF016A GM Vehicle Speed Arbitration)' '#154' 'true' 'REQ:  154' '' } %GIDa_ed2c8f3b_0ba1_4891_b977_6af525739620"
  VehSpdMinSecurVld : Outport  RequirementInfo="{'linktype_rmi_doors' '0000c6e6 (/GM T1XX/SubSystem Specifications/Customer Functions/CF016A GM Vehicle Speed Arbitration)' '#200' 'true' 'REQ:  200' '' } %GIDa_e167b267_07d4_4cec_a018_d9eb5601378f"  Port=2
  wires:
  Constant3/1 -> VehSpdMinSecurVld/1
  If3/1 -> Min_LeNonDrvnBusHiSpd_LeNonDrvnBusChassisExp/Action
  If3/2 -> Set_VehSpdMinSecur_Max/Action
  If18/1 -> Get_Min/Action
  If18/2 -> Pass_VehSpdMinSecur/Action
  Min_LeNonDrvnBusHiSpd_LeNonDrvnBusChassisExp/1(TmpMinSpd) -> Merge26/1
  Set_VehSpdMinSecur_Max/1(TmpMinSpd) -> Merge26/2
  Pass_VehSpdMinSecur/1(TmpMinSpd) -> Merge28/2
  Get_Min/1(TmpMinSpd) -> Merge28/1
  LeNonDrvnVld/1 -> If3/1
  RiNonDrvnVld/1 -> If18/1
  RiNonDrvnBusChassisExp/1 -> Get_Min/2(RiNonDrvnBusChassisExp)
  RiNonDrvnBusHiSpd/1 -> Get_Min/3(RiNonDrvnBusHiSpd)
  Merge26/1 -> [TmpVehSpdMinSecur], Pass_VehSpdMinSecur/1(TmpVehSpdMinSecur)
  [TmpVehSpdMinSecur] -> Get_Min/1(TmpVehSpdMinSecur)
  Merge28/1 -> VehSpdMinSecur/1  "TmpMinSpd_Kph_T_f32"
  LeNonDrvnBusHiSpd/1 -> Min_LeNonDrvnBusHiSpd_LeNonDrvnBusChassisExp/1(LeNonDrvnBusHiSpd)
  LeNonDrvnBusChassisExp/1 -> Min_LeNonDrvnBusHiSpd_LeNonDrvnBusChassisExp/2(LeNonDrvnBusChassisExp)
  Constant1/1 -> Set_VehSpdMinSecur_Max/1(TmpVehSpdMinSecur)

== system CF016A_GmVehSpdArbn/GmVehSpdArbn/GmVehSpdArbnPer1/CopyRight2 ==

== system CF016A_GmVehSpdArbn/GmVehSpdArbn/GmVehSpdArbnPer1/LeDrvnVld ==
  RawSignalMux : Inport  RequirementInfo="{'linktype_rmi_doors' '0000c6e6 (/GM T1XX/SubSystem Specifications/Customer Functions/CF016A GM Vehicle Speed Arbitration)' '#134' 'true' 'REQ:  134' '' } %GIDa_850fbadf_899f_4ef0_a1ec_0c685cc62edd"
  CopyRight2 : Subsystem  Description=|  RequirementInfo="{'linktype_rmi_doors' '0000c6e6 (/GM T1XX/SubSystem Specifications/Customer Functions/CF016A GM Vehicle Speed Arbitration)' '#134' 'true' 'REQ:  134' '' } %GIDa_67058dd0_604b_48fc_9a7a_ff0a59654575"  mask(Copyright Information){none=on}
      | Copyright info block.                                               
      |                                                                     
      | Place copyright information at the top of every subsystem in design.
      mask prompts: none "No parameters"
      mask help: Place copyright information at the top of every subsystem in design.
      mask Display:
      | NxtrConf = 'Nexteer Confidential';
      | 
      | sys = bdroot; %handle for the current model ("system")
      | first = get_param(sys,'Created');
      | if(isempty(first))
      |     first = datestr(now,'yyyy');
      | else
      |     first = first(end-3:end);  %year is last four digits
      | end
      | 
      | last = get_param(sys,'LastModifiedDate');
      | if isempty(last)
      |     last = datestr(now,'yyyy');
      | else
      |     last = last(end-3:end);
      | end
      | 
      | if strcmp(first,last)
      |     fprintf('%s -- Copyright %s Nexteer',NxtrConf,first)
      | else
      |     fprintf('%s -- %s%s- %s Nexteer',NxtrConf,char(169),first,last)
      | end
  Demux : Demux  RequirementInfo="{'linktype_rmi_doors' '0000c6e6 (/GM T1XX/SubSystem Specifications/Customer Functions/CF016A GM Vehicle Speed Arbitration)' '#134' 'true' 'REQ:  134' '' } %GIDa_d9942494_8589_4348_9113_3fe4093ccc1e"
  LeDrvnVld_IF : If  RequirementInfo="{'linktype_rmi_doors' '0000c6e6 (/GM T1XX/SubSystem Specifications/Customer Functions/CF016A GM Vehicle Speed Arbitration)' '#134' 'true' 'REQ:  134' '' } %GIDa_52b48005_83ac_43c9_90d8_0785c8fc7ba6"  NumInputs=4  IfExpression=~u1|u2|u3|(~u4)
      settings: AttributesFormatString=%<Priority>
  Merge1 : Merge  RequirementInfo="{'linktype_rmi_doors' '0000c6e6 (/GM T1XX/SubSystem Specifications/Customer Functions/CF016A GM Vehicle Speed Arbitration)' '#134' 'true' 'REQ:  134' '' } %GIDa_eae018c6_c4a7_4658_9413_f070945a9b23"
  Set_LeDrvnVld_False : Subsystem  RequirementInfo="{'linktype_rmi_doors' '0000c6e6 (/GM T1XX/SubSystem Specifications/Customer Functions/CF016A GM Vehicle Speed Arbitration)' '#134' 'true' 'REQ:  134' '' } %GIDa_3f6bd0c0_9e75_409f_b8bc_6260bb2dac5d"  TreatAsAtomicUnit=on
  Set_LeDrvnVld_True : Subsystem  RequirementInfo="{'linktype_rmi_doors' '0000c6e6 (/GM T1XX/SubSystem Specifications/Customer Functions/CF016A GM Vehicle Speed Arbitration)' '#134' 'true' 'REQ:  134' '' } %GIDa_7501a4e8_44e8_4b43_bcf9_2cb5f06d8c29"  TreatAsAtomicUnit=on
  LeDrvnVld : Outport  RequirementInfo="{'linktype_rmi_doors' '0000c6e6 (/GM T1XX/SubSystem Specifications/Customer Functions/CF016A GM Vehicle Speed Arbitration)' '#134' 'true' 'REQ:  134' '' } %GIDa_8357c082_e1ff_4eba_b727_33f4d045b639"
  wires:
  LeDrvnVld_IF/2 -> Set_LeDrvnVld_True/Action
  LeDrvnVld_IF/1 -> Set_LeDrvnVld_False/Action
  Set_LeDrvnVld_False/1(LeDrvnVld) -> Merge1/1
  Set_LeDrvnVld_True/1(LeDrvnVld) -> Merge1/2
  Merge1/1 -> LeDrvnVld/1  "LeDrvnVld_Cnt_T_logl"
  RawSignalMux/1 -> Demux/1
  Demux/1 -> LeDrvnVld_IF/1
  Demux/2 -> LeDrvnVld_IF/2
  Demux/3 -> LeDrvnVld_IF/3
  Demux/4 -> LeDrvnVld_IF/4

== system CF016A_GmVehSpdArbn/GmVehSpdArbn/GmVehSpdArbnPer1/LeNonDrvnVld ==
  RawSignalMux : Inport  RequirementInfo="{'linktype_rmi_doors' '0000c6e6 (/GM T1XX/SubSystem Specifications/Customer Functions/CF016A GM Vehicle Speed Arbitration)' '#164' 'true' 'REQ:  164' '' } %GIDa_06872a1b_d038_44fc_b8ba_c3e4b180c86a"
  CopyRight2 : Subsystem  Description=|  RequirementInfo="{'linktype_rmi_doors' '0000c6e6 (/GM T1XX/SubSystem Specifications/Customer Functions/CF016A GM Vehicle Speed Arbitration)' '#164' 'true' 'REQ:  164' '' } %GIDa_17f1ba1d_dd62_4b8a_81a2_959252fd4e8a"  mask(Copyright Information){none=on}
      | Copyright info block.                                               
      |                                                                     
      | Place copyright information at the top of every subsystem in design.
      mask prompts: none "No parameters"
      mask help: Place copyright information at the top of every subsystem in design.
      mask Display:
      | NxtrConf = 'Nexteer Confidential';
      | 
      | sys = bdroot; %handle for the current model ("system")
      | first = get_param(sys,'Created');
      | if(isempty(first))
      |     first = datestr(now,'yyyy');
      | else
      |     first = first(end-3:end);  %year is last four digits
      | end
      | 
      | last = get_param(sys,'LastModifiedDate');
      | if isempty(last)
      |     last = datestr(now,'yyyy');
      | else
      |     last = last(end-3:end);
      | end
      | 
      | if strcmp(first,last)
      |     fprintf('%s -- Copyright %s Nexteer',NxtrConf,first)
      | else
      |     fprintf('%s -- %s%s- %s Nexteer',NxtrConf,char(169),first,last)
      | end
  Demux : Demux  RequirementInfo="{'linktype_rmi_doors' '0000c6e6 (/GM T1XX/SubSystem Specifications/Customer Functions/CF016A GM Vehicle Speed Arbitration)' '#164' 'true' 'REQ:  164' '' } %GIDa_45672ca2_6ef5_46c8_b9d3_d0e7e64ea7d1"
  LeNonDrvnVld_IF : If  RequirementInfo="{'linktype_rmi_doors' '0000c6e6 (/GM T1XX/SubSystem Specifications/Customer Functions/CF016A GM Vehicle Speed Arbitration)' '#164' 'true' 'REQ:  164' '' } %GIDa_c24ece7c_8b02_4a05_a8e9_ca42574ee183"  NumInputs=4  IfExpression=~u1|u2|u3| ~u4
      settings: AttributesFormatString=%<Priority>
  Merge3 : Merge  RequirementInfo="{'linktype_rmi_doors' '0000c6e6 (/GM T1XX/SubSystem Specifications/Customer Functions/CF016A GM Vehicle Speed Arbitration)' '#164' 'true' 'REQ:  164' '' } %GIDa_32c8c45c_8dce_4270_a845_63368eceb542"
  Set_LeNonDrvnVld_False : Subsystem  RequirementInfo="{'linktype_rmi_doors' '0000c6e6 (/GM T1XX/SubSystem Specifications/Customer Functions/CF016A GM Vehicle Speed Arbitration)' '#164' 'true' 'REQ:  164' '' } %GIDa_c6498d04_a6e9_4924_a9b3_67c7d95ed469"  TreatAsAtomicUnit=on
  Set_LeNonDrvnVld_True : Subsystem  RequirementInfo="{'linktype_rmi_doors' '0000c6e6 (/GM T1XX/SubSystem Specifications/Customer Functions/CF016A GM Vehicle Speed Arbitration)' '#164' 'true' 'REQ:  164' '' } %GIDa_324b2528_1be5_4d0d_a4d7_794f8b7e728d"  TreatAsAtomicUnit=on
  LeNonDrvnVld : Outport  RequirementInfo="{'linktype_rmi_doors' '0000c6e6 (/GM T1XX/SubSystem Specifications/Customer Functions/CF016A GM Vehicle Speed Arbitration)' '#164' 'true' 'REQ:  164' '' } %GIDa_e1163ca8_f447_4093_b5bf_c8228f3aba4a"
  wires:
  LeNonDrvnVld_IF/2 -> Set_LeNonDrvnVld_True/Action
  LeNonDrvnVld_IF/1 -> Set_LeNonDrvnVld_False/Action
  Set_LeNonDrvnVld_False/1(LeNonDrvnVld) -> Merge3/1
  Set_LeNonDrvnVld_True/1(LeNonDrvnVld) -> Merge3/2
  Merge3/1 -> LeNonDrvnVld/1  "LeNonDrvnVld_Cnt_T_logl"
  RawSignalMux/1 -> Demux/1
  Demux/1 -> LeNonDrvnVld_IF/1
  Demux/2 -> LeNonDrvnVld_IF/2
  Demux/3 -> LeNonDrvnVld_IF/3
  Demux/4 -> LeNonDrvnVld_IF/4

== system CF016A_GmVehSpdArbn/GmVehSpdArbn/GmVehSpdArbnPer1/RiDrvnVld ==
  RawSignalMux : Inport  RequirementInfo="{'linktype_rmi_doors' '0000c6e6 (/GM T1XX/SubSystem Specifications/Customer Functions/CF016A GM Vehicle Speed Arbitration)' '#148' 'true' 'REQ:  148' '' } %GIDa_8c3ed26a_7e3c_4a6b_9d36_8fb1fc4a1b03"
  CopyRight2 : Subsystem  Description=|  RequirementInfo="{'linktype_rmi_doors' '0000c6e6 (/GM T1XX/SubSystem Specifications/Customer Functions/CF016A GM Vehicle Speed Arbitration)' '#148' 'true' 'REQ:  148' '' } %GIDa_902af99a_cc88_4079_9b25_29116fcd4e52"  mask(Copyright Information){none=on}
      | Copyright info block.                                               
      |                                                                     
      | Place copyright information at the top of every subsystem in design.
      mask prompts: none "No parameters"
      mask help: Place copyright information at the top of every subsystem in design.
      mask Display:
      | NxtrConf = 'Nexteer Confidential';
      | 
      | sys = bdroot; %handle for the current model ("system")
      | first = get_param(sys,'Created');
      | if(isempty(first))
      |     first = datestr(now,'yyyy');
      | else
      |     first = first(end-3:end);  %year is last four digits
      | end
      | 
      | last = get_param(sys,'LastModifiedDate');
      | if isempty(last)
      |     last = datestr(now,'yyyy');
      | else
      |     last = last(end-3:end);
      | end
      | 
      | if strcmp(first,last)
      |     fprintf('%s -- Copyright %s Nexteer',NxtrConf,first)
      | else
      |     fprintf('%s -- %s%s- %s Nexteer',NxtrConf,char(169),first,last)
      | end
  Demux : Demux  RequirementInfo="{'linktype_rmi_doors' '0000c6e6 (/GM T1XX/SubSystem Specifications/Customer Functions/CF016A GM Vehicle Speed Arbitration)' '#148' 'true' 'REQ:  148' '' } %GIDa_ddf3d15b_b217_4527_bd9a_9d08b962ee30"
  Merge2 : Merge  RequirementInfo="{'linktype_rmi_doors' '0000c6e6 (/GM T1XX/SubSystem Specifications/Customer Functions/CF016A GM Vehicle Speed Arbitration)' '#148' 'true' 'REQ:  148' '' } %GIDa_80e61bf6_614a_400f_96e9_9365f94bfaf9"
  RiDrvnVld_IF : If  RequirementInfo="{'linktype_rmi_doors' '0000c6e6 (/GM T1XX/SubSystem Specifications/Customer Functions/CF016A GM Vehicle Speed Arbitration)' '#148' 'true' 'REQ:  148' '' } %GIDa_83cf1c79_b38b_458e_802a_741953ce747e"  NumInputs=4  IfExpression=~u1|u2|u3|(~u4)
      settings: AttributesFormatString=%<Priority>
  Set_RiDrvnVld_False : Subsystem  RequirementInfo="{'linktype_rmi_doors' '0000c6e6 (/GM T1XX/SubSystem Specifications/Customer Functions/CF016A GM Vehicle Speed Arbitration)' '#148' 'true' 'REQ:  148' '' } %GIDa_77d7a8a4_f259_40fb_aee5_afd2c04b13cf"  TreatAsAtomicUnit=on
  Set_RiDrvnVld_True : Subsystem  RequirementInfo="{'linktype_rmi_doors' '0000c6e6 (/GM T1XX/SubSystem Specifications/Customer Functions/CF016A GM Vehicle Speed Arbitration)' '#148' 'true' 'REQ:  148' '' } %GIDa_85287ead_3864_4722_b883_88f96053c235"  TreatAsAtomicUnit=on
  RiDrvnVld : Outport  RequirementInfo="{'linktype_rmi_doors' '0000c6e6 (/GM T1XX/SubSystem Specifications/Customer Functions/CF016A GM Vehicle Speed Arbitration)' '#148' 'true' 'REQ:  148' '' } %GIDa_f81d9b1c_8811_4a67_a358_4719dd0e5a0d"
  wires:
  RiDrvnVld_IF/2 -> Set_RiDrvnVld_True/Action
  RiDrvnVld_IF/1 -> Set_RiDrvnVld_False/Action
  Set_RiDrvnVld_False/1(RiDrvnVld) -> Merge2/1
  Set_RiDrvnVld_True/1(RiDrvnVld) -> Merge2/2
  Merge2/1 -> RiDrvnVld/1  "RiDrvnVld_Cnt_T_logl"
  RawSignalMux/1 -> Demux/1
  Demux/1 -> RiDrvnVld_IF/1
  Demux/2 -> RiDrvnVld_IF/2
  Demux/3 -> RiDrvnVld_IF/3
  Demux/4 -> RiDrvnVld_IF/4

== system CF016A_GmVehSpdArbn/GmVehSpdArbn/GmVehSpdArbnPer1/RiNonDrvnVld ==
  RawSignalMux : Inport  RequirementInfo="{'linktype_rmi_doors' '0000c6e6 (/GM T1XX/SubSystem Specifications/Customer Functions/CF016A GM Vehicle Speed Arbitration)' '#165' 'true' 'REQ:  165' '' } %GIDa_0f61b8d2_2e12_4891_a383_5ee44243ae32"
  CopyRight2 : Subsystem  Description=|  RequirementInfo="{'linktype_rmi_doors' '0000c6e6 (/GM T1XX/SubSystem Specifications/Customer Functions/CF016A GM Vehicle Speed Arbitration)' '#165' 'true' 'REQ:  165' '' } %GIDa_8d625cc7_052c_42ec_8855_b93ea657090f"  mask(Copyright Information){none=on}
      | Copyright info block.                                               
      |                                                                     
      | Place copyright information at the top of every subsystem in design.
      mask prompts: none "No parameters"
      mask help: Place copyright information at the top of every subsystem in design.
      mask Display:
      | NxtrConf = 'Nexteer Confidential';
      | 
      | sys = bdroot; %handle for the current model ("system")
      | first = get_param(sys,'Created');
      | if(isempty(first))
      |     first = datestr(now,'yyyy');
      | else
      |     first = first(end-3:end);  %year is last four digits
      | end
      | 
      | last = get_param(sys,'LastModifiedDate');
      | if isempty(last)
      |     last = datestr(now,'yyyy');
      | else
      |     last = last(end-3:end);
      | end
      | 
      | if strcmp(first,last)
      |     fprintf('%s -- Copyright %s Nexteer',NxtrConf,first)
      | else
      |     fprintf('%s -- %s%s- %s Nexteer',NxtrConf,char(169),first,last)
      | end
  Demux : Demux  RequirementInfo="{'linktype_rmi_doors' '0000c6e6 (/GM T1XX/SubSystem Specifications/Customer Functions/CF016A GM Vehicle Speed Arbitration)' '#165' 'true' 'REQ:  165' '' } %GIDa_6645711b_9486_464d_a81d_8f7e7bd5c37f"
  Merge4 : Merge  RequirementInfo="{'linktype_rmi_doors' '0000c6e6 (/GM T1XX/SubSystem Specifications/Customer Functions/CF016A GM Vehicle Speed Arbitration)' '#165' 'true' 'REQ:  165' '' } %GIDa_227b30f1_55a5_415b_8714_8d470ac92be4"
  RiNonDrvnVld_IF : If  RequirementInfo="{'linktype_rmi_doors' '0000c6e6 (/GM T1XX/SubSystem Specifications/Customer Functions/CF016A GM Vehicle Speed Arbitration)' '#165' 'true' 'REQ:  165' '' } %GIDa_8c1d2cf5_e5ee_4c1a_b2ba_c7b94cb354b6"  NumInputs=4  IfExpression=~u1|u2|u3| ~u4
      settings: AttributesFormatString=%<Priority>
  Set_RiNonDrvnVld_False : Subsystem  RequirementInfo="{'linktype_rmi_doors' '0000c6e6 (/GM T1XX/SubSystem Specifications/Customer Functions/CF016A GM Vehicle Speed Arbitration)' '#165' 'true' 'REQ:  165' '' } %GIDa_8e47a6da_e28e_4013_9480_de94ca63738b"  TreatAsAtomicUnit=on
  Set_RiNonDrvnVld_True : Subsystem  RequirementInfo="{'linktype_rmi_doors' '0000c6e6 (/GM T1XX/SubSystem Specifications/Customer Functions/CF016A GM Vehicle Speed Arbitration)' '#165' 'true' 'REQ:  165' '' } %GIDa_7ab08d59_8551_49e6_af86_df6fda3c6b91"  TreatAsAtomicUnit=on
  RiNonDrvnVld : Outport  RequirementInfo="{'linktype_rmi_doors' '0000c6e6 (/GM T1XX/SubSystem Specifications/Customer Functions/CF016A GM Vehicle Speed Arbitration)' '#165' 'true' 'REQ:  165' '' } %GIDa_72540e04_d2bd_46dd_b773_51e13bfb89b0"
  wires:
  RiNonDrvnVld_IF/2 -> Set_RiNonDrvnVld_True/Action
  RiNonDrvnVld_IF/1 -> Set_RiNonDrvnVld_False/Action
  Set_RiNonDrvnVld_False/1(RiNonDrvnVld) -> Merge4/1
  Set_RiNonDrvnVld_True/1(RiNonDrvnVld) -> Merge4/2
  Merge4/1 -> RiNonDrvnVld/1  "RiNonDrvnVld_Cnt_T_logl"
  RawSignalMux/1 -> Demux/1
  Demux/1 -> RiNonDrvnVld_IF/1
  Demux/2 -> RiNonDrvnVld_IF/2
  Demux/3 -> RiNonDrvnVld_IF/3
  Demux/4 -> RiNonDrvnVld_IF/4
